simulink model "Machine_synchrone"  (R2016a)
settings: Solver=VariableStepAuto  StartTime=0.0  StopTime=0.3  RelTol=1e-3
values from neighbouring files (symbols this model uses):
  Kid = 3/(Td*kd)    (= 16502.7862857)    [Data.m]
  Kiq = 3/(Tq*kq)    (= 9368.0205239)    [Data.m]
  Pd = 3/kd    (= 38.6928)    [Data.m]
  Pq = 3/kq    (= 34.3565217391)    [Data.m]
libraries: cstblocks x2
settings Model: Creator=NAD  LastModifiedBy=NAD

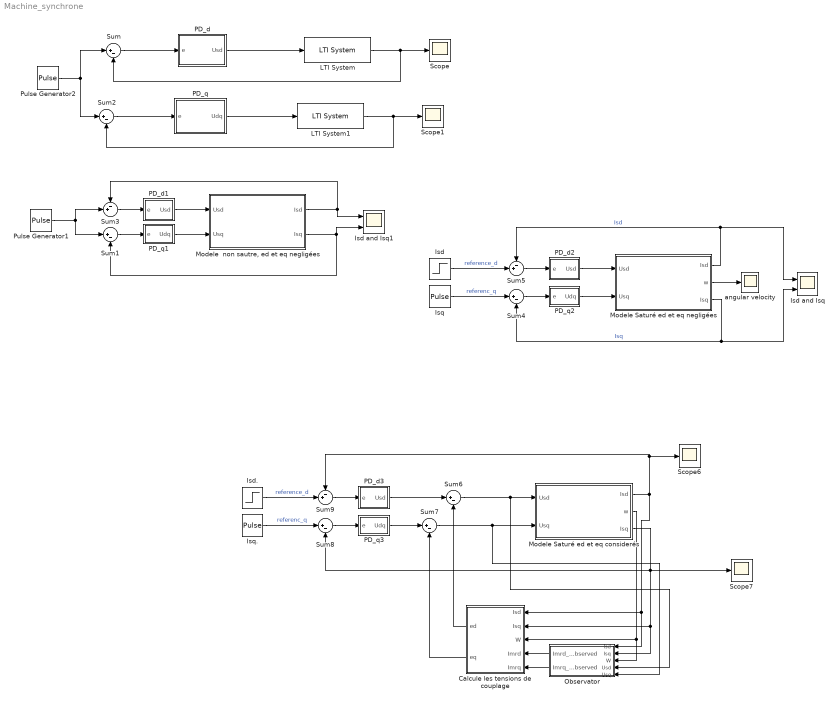
== system Machine_synchrone ==
  Calcule les tensions de couplage : MATLAB Function  TreatAsAtomicUnit=on
  Isd : Step  Time=0  After=10  SampleTime=0
  Isd and Isq : Scope  NumInputPorts=2
  Isd and Isq1 : Scope  NumInputPorts=2
  Isd. : Step  Time=0  After=10  SampleTime=0
  Isq : DiscretePulseGenerator  PulseType=Time based  Amplitude=10  Period=0.2  PulseWidth=50
  Isq. : DiscretePulseGenerator  PulseType=Time based  Amplitude=10  Period=0.2  PulseWidth=50
  LTI System : cstblocks/LTI System  sys=Fd  IC=[]
  LTI System1 : cstblocks/LTI System  sys=Fq  IC=[]
  "Modele  non sautre, ed et eq negligées" : Subsystem
  Modele Saturé ed et eq considerés : Subsystem
  Modele Saturé ed et eq negligées : Subsystem
  Observator : Subsystem
  PD_d : Subsystem
  PD_d1 : Subsystem
  PD_d2 : Subsystem
  PD_d3 : Subsystem
  PD_q : Subsystem
  PD_q1 : Subsystem
  PD_q2 : Subsystem
  PD_q3 : Subsystem
  Pulse Generator1 : DiscretePulseGenerator  PulseType=Time based  Amplitude=10  Period=1  PulseWidth=50
  Pulse Generator2 : DiscretePulseGenerator  PulseType=Time based  Amplitude=5  Period=0.01  PulseWidth=50
  Scope{,1,6..7} (4 alike) : Scope
  Sum{,1..2,4,6..8} (7 alike) : Sum  Inputs=|+-
  Sum3 : Sum  Inputs=-+|
  Sum5 : Sum  Inputs=-+|
  Sum9 : Sum  Inputs=-+|
  angular velocity : Scope
  wires:
  LTI System/1 -> Scope/1, Sum/2
  LTI System1/1 -> Scope1/1, Sum2/2
  Sum/1 -> PD_d/1(e)
  PD_d/1(Usd) -> LTI System/1
  Sum2/1 -> PD_q/1(e)
  PD_q/1(Udq) -> LTI System1/1
  PD_d1/1(Usd) -> "Modele  non sautre, ed et eq negligées"/1(Usd)
  PD_q1/1(Udq) -> "Modele  non sautre, ed et eq negligées"/2(Usq)
  "Modele  non sautre, ed et eq negligées"/1(Isd) -> Sum3/1, Isd and Isq1/1
  "Modele  non sautre, ed et eq negligées"/2(Isq) -> Sum1/2, Isd and Isq1/2
  Sum1/1 -> PD_q1/1(e)
  Sum3/1 -> PD_d1/1(e)
  Pulse Generator1/1 -> Sum3/2, Sum1/1
  PD_d2/1(Usd) -> Modele Saturé ed et eq negligées/1(Usd)
  PD_q2/1(Udq) -> Modele Saturé ed et eq negligées/2(Usq)
  Modele Saturé ed et eq negligées/1(Isd) -> Isd and Isq/1, Sum5/1  "Isd"
  Sum4/1 -> PD_q2/1(e)
  Sum5/1 -> PD_d2/1(e)
  Isq/1 -> Sum4/1  "referenc_q"
  Modele Saturé ed et eq negligées/3(Isq) -> Isd and Isq/2, Sum4/2  "Isq"
  Sum6/1 -> Observator/4(Usd), Modele Saturé ed et eq considerés/1(Usd)
  Sum7/1 -> Observator/5(Usq), Modele Saturé ed et eq considerés/2(Usq)
  Modele Saturé ed et eq considerés/1(Isd) -> Scope6/1, Sum9/1, Calcule les tensions de couplage/1(Isd), Observator/1(Isd)
  Sum8/1 -> PD_q3/1(e)
  Sum9/1 -> PD_d3/1(e)
  Modele Saturé ed et eq considerés/3(Isq) -> Calcule les tensions de couplage/2(Isq), Observator/2(Isq), Scope7/1, Sum8/2
  Observator/1(Imrd_Observed) -> Calcule les tensions de couplage/4(Imrd)
  Observator/2(Imrq_Observed) -> Calcule les tensions de couplage/5(Imrq)
  Modele Saturé ed et eq considerés/2(w) -> Calcule les tensions de couplage/3(W), Observator/3(W)
  Calcule les tensions de couplage/1(ed) -> Sum6/2
  Calcule les tensions de couplage/2(eq) -> Sum7/2
  PD_q3/1(Udq) -> Sum7/1
  PD_d3/1(Usd) -> Sum6/1
  Pulse Generator2/1 -> Sum/1, Sum2/1
  Modele Saturé ed et eq negligées/2(w) -> angular velocity/1
  Isd/1 -> Sum5/2  "reference_d"
  Isq./1 -> Sum8/1  "referenc_q"
  Isd./1 -> Sum9/2  "reference_d"

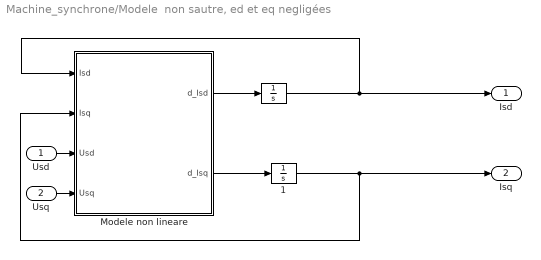
== system Machine_synchrone/Modele  non sautre, ed et eq negligées ==
  Usd : Inport
  Usq : Inport  Port=2
  " " : Integrator
  " 1" : Integrator
  Modele non lineare : MATLAB Function  TreatAsAtomicUnit=on
  Isd : Outport
  Isq : Outport  Port=2
  wires:
  Modele non lineare/2(d_Isq) -> " 1"/1
  " 1"/1 -> Isq/1, Modele non lineare/2(Isq)
  Usq/1 -> Modele non lineare/4(Usq)
  Usd/1 -> Modele non lineare/3(Usd)
  Modele non lineare/1(d_Isd) -> " "/1
  " "/1 -> Modele non lineare/1(Isd), Isd/1

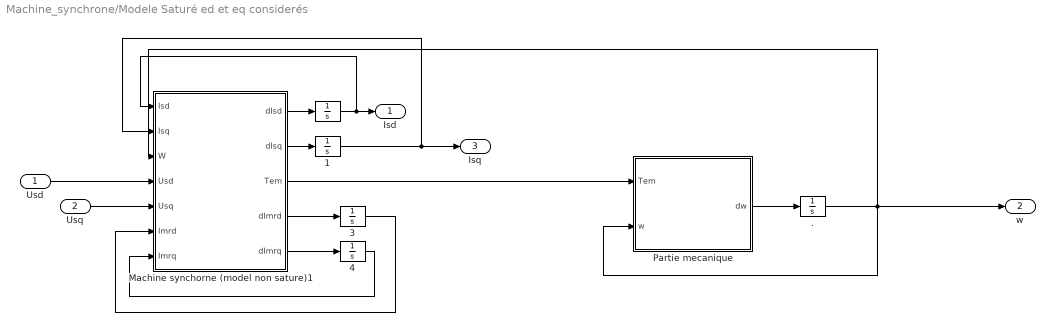
== system Machine_synchrone/Modele Saturé ed et eq considerés ==
  Usd : Inport
  Usq : Inport  Port=2
  " " : Integrator
  " ." : Integrator
  " 1" : Integrator
  " 3" : Integrator  InitialCondition=0.01
  " 4" : Integrator  InitialCondition=0.01
  Machine synchorne (model non sature)1 : MATLAB Function  TreatAsAtomicUnit=on
  Partie mecanique : MATLAB Function  TreatAsAtomicUnit=on
  Isd : Outport
  w : Outport  Port=2
  Isq : Outport  Port=3
  wires:
  " 3"/1 -> Machine synchorne (model non sature)1/6(Imrd)
  " 4"/1 -> Machine synchorne (model non sature)1/7(Imrq)
  Machine synchorne (model non sature)1/5(dImrq) -> " 4"/1
  Machine synchorne (model non sature)1/4(dImrd) -> " 3"/1
  Usq/1 -> Machine synchorne (model non sature)1/5(Usq)
  Usd/1 -> Machine synchorne (model non sature)1/4(Usd)
  " 1"/1 -> Isq/1, Machine synchorne (model non sature)1/2(Isq)
  Machine synchorne (model non sature)1/2(dIsq) -> " 1"/1
  Machine synchorne (model non sature)1/3(Tem) -> Partie mecanique/1(Tem)
  Partie mecanique/1(dw) -> " ."/1
  " ."/1 -> Machine synchorne (model non sature)1/3(W), Partie mecanique/2(w), w/1
  " "/1 -> Machine synchorne (model non sature)1/1(Isd), Isd/1
  Machine synchorne (model non sature)1/1(dIsd) -> " "/1

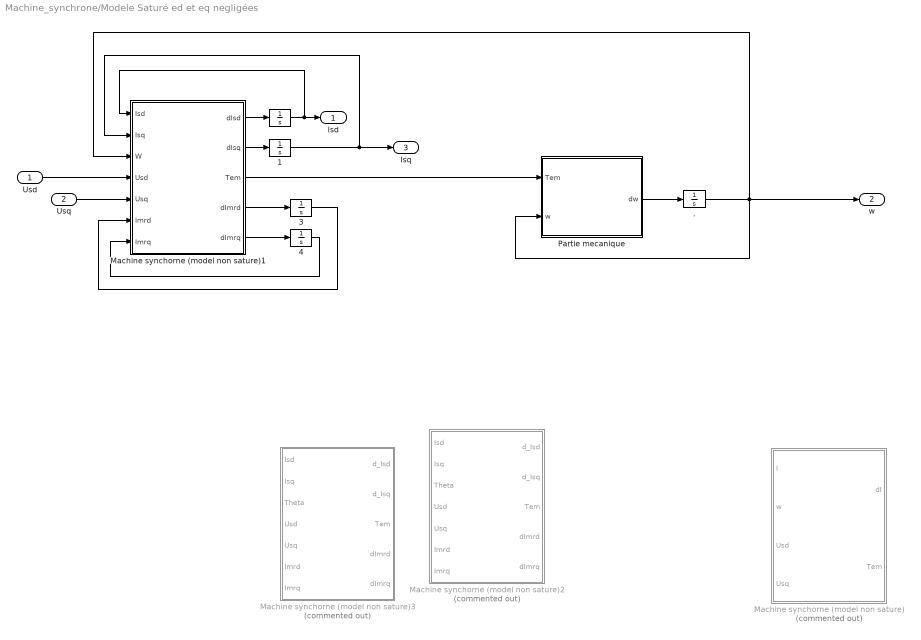
== system Machine_synchrone/Modele Saturé ed et eq negligées ==
  Usd : Inport
  Usq : Inport  Port=2
  " " : Integrator
  " ." : Integrator
  " 1" : Integrator
  " 3" : Integrator  InitialCondition=0.01
  " 4" : Integrator  InitialCondition=0.01
  Machine synchorne (model non sature) : MATLAB Function  Commented=on  TreatAsAtomicUnit=on
  Machine synchorne (model non sature)1 : MATLAB Function  TreatAsAtomicUnit=on
  Machine synchorne (model non sature)2 : MATLAB Function  Commented=on  TreatAsAtomicUnit=on
  Machine synchorne (model non sature)3 : MATLAB Function  Commented=on  TreatAsAtomicUnit=on
  Partie mecanique : MATLAB Function  TreatAsAtomicUnit=on
  Isd : Outport
  w : Outport  Port=2
  Isq : Outport  Port=3
  wires:
  Machine synchorne (model non sature)1/1(dIsd) -> " "/1
  " "/1 -> Isd/1, Machine synchorne (model non sature)1/1(Isd)
  " ."/1 -> w/1, Partie mecanique/2(w), Machine synchorne (model non sature)1/3(W)
  Partie mecanique/1(dw) -> " ."/1
  Machine synchorne (model non sature)1/3(Tem) -> Partie mecanique/1(Tem)
  Machine synchorne (model non sature)1/2(dIsq) -> " 1"/1
  " 1"/1 -> Machine synchorne (model non sature)1/2(Isq), Isq/1
  Usd/1 -> Machine synchorne (model non sature)1/4(Usd)
  Usq/1 -> Machine synchorne (model non sature)1/5(Usq)
  Machine synchorne (model non sature)1/4(dImrd) -> " 3"/1
  Machine synchorne (model non sature)1/5(dImrq) -> " 4"/1
  " 4"/1 -> Machine synchorne (model non sature)1/7(Imrq)
  " 3"/1 -> Machine synchorne (model non sature)1/6(Imrd)

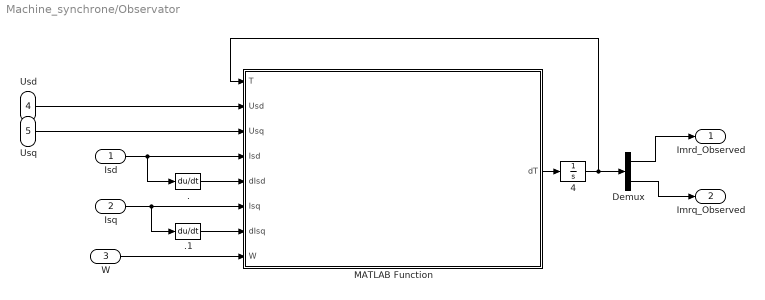
== system Machine_synchrone/Observator ==
  Isd : Inport
  Isq : Inport  Port=2
  W : Inport  Port=3
  Usd : Inport  Port=4
  Usq : Inport  Port=5
  " 4" : Integrator  InitialCondition=0.01*[1;1]
  . : Derivative
  .1 : Derivative
  Demux : Demux  Outputs=2
  MATLAB Function : MATLAB Function  TreatAsAtomicUnit=on
  Imrd_Observed : Outport
  Imrq_Observed : Outport  Port=2
  wires:
  W/1 -> MATLAB Function/8(W)
  .1/1 -> MATLAB Function/7(dIsq)
  MATLAB Function/1(dT) -> " 4"/1
  " 4"/1 -> Demux/1, MATLAB Function/1(T)
  ./1 -> MATLAB Function/5(dIsd)
  Demux/1 -> Imrd_Observed/1
  Isq/1 -> .1/1, MATLAB Function/6(Isq)
  Isd/1 -> MATLAB Function/4(Isd), ./1
  Usd/1 -> MATLAB Function/2(Usd)
  Demux/2 -> Imrq_Observed/1
  Usq/1 -> MATLAB Function/3(Usq)

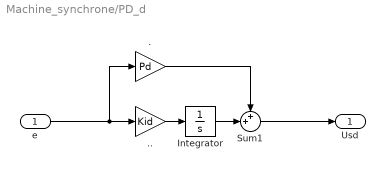
== system Machine_synchrone/PD_d ==
  e : Inport
  ". " : Gain  Gain=Pd
  .. : Gain  Gain=Kid
  Integrator : Integrator
  Sum1 : Sum  Inputs=++|
  Usd : Outport
  wires:
  Sum1/1 -> Usd/1
  e/1 -> ../1, ". "/1
  ". "/1 -> Sum1/1
  Integrator/1 -> Sum1/2
  ../1 -> Integrator/1

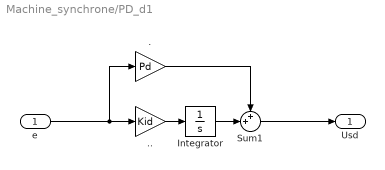
== system Machine_synchrone/PD_d1 ==
  e : Inport
  ". " : Gain  Gain=Pd
  .. : Gain  Gain=Kid
  Integrator : Integrator
  Sum1 : Sum  Inputs=++|
  Usd : Outport
  wires:
  ../1 -> Integrator/1
  Integrator/1 -> Sum1/2
  ". "/1 -> Sum1/1
  e/1 -> ". "/1, ../1
  Sum1/1 -> Usd/1

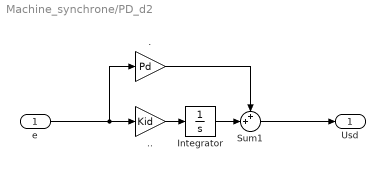
== system Machine_synchrone/PD_d2 ==
  e : Inport
  ". " : Gain  Gain=Pd
  .. : Gain  Gain=Kid
  Integrator : Integrator
  Sum1 : Sum  Inputs=++|
  Usd : Outport
  wires:
  ../1 -> Integrator/1
  Integrator/1 -> Sum1/2
  ". "/1 -> Sum1/1
  e/1 -> ". "/1, ../1
  Sum1/1 -> Usd/1

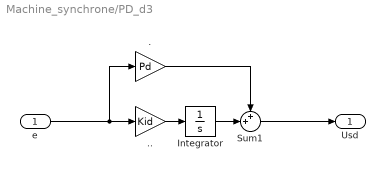
== system Machine_synchrone/PD_d3 ==
  e : Inport
  ". " : Gain  Gain=Pd
  .. : Gain  Gain=Kid
  Integrator : Integrator
  Sum1 : Sum  Inputs=++|
  Usd : Outport
  wires:
  Sum1/1 -> Usd/1
  e/1 -> ../1, ". "/1
  ". "/1 -> Sum1/1
  Integrator/1 -> Sum1/2
  ../1 -> Integrator/1

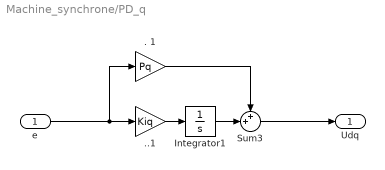
== system Machine_synchrone/PD_q ==
  e : Inport
  . 1 : Gain  Gain=Pq
  ..1 : Gain  Gain=Kiq
  Integrator1 : Integrator
  Sum3 : Sum  Inputs=++|
  Udq : Outport
  wires:
  Sum3/1 -> Udq/1
  Integrator1/1 -> Sum3/2
  . 1/1 -> Sum3/1
  e/1 -> . 1/1, ..1/1
  ..1/1 -> Integrator1/1

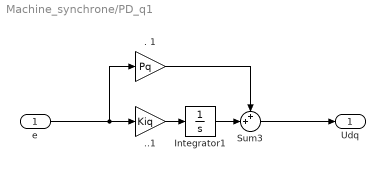
== system Machine_synchrone/PD_q1 ==
  e : Inport
  . 1 : Gain  Gain=Pq
  ..1 : Gain  Gain=Kiq
  Integrator1 : Integrator
  Sum3 : Sum  Inputs=++|
  Udq : Outport
  wires:
  ..1/1 -> Integrator1/1
  e/1 -> ..1/1, . 1/1
  . 1/1 -> Sum3/1
  Integrator1/1 -> Sum3/2
  Sum3/1 -> Udq/1

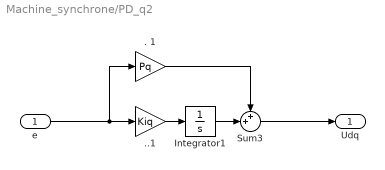
== system Machine_synchrone/PD_q2 ==
  e : Inport
  . 1 : Gain  Gain=Pq
  ..1 : Gain  Gain=Kiq
  Integrator1 : Integrator
  Sum3 : Sum  Inputs=++|
  Udq : Outport
  wires:
  ..1/1 -> Integrator1/1
  e/1 -> ..1/1, . 1/1
  . 1/1 -> Sum3/1
  Integrator1/1 -> Sum3/2
  Sum3/1 -> Udq/1

== system Machine_synchrone/PD_q3 ==
  e : Inport
  . 1 : Gain  Gain=Pq
  ..1 : Gain  Gain=Kiq
  Integrator1 : Integrator
  Sum3 : Sum  Inputs=++|
  Udq : Outport
  wires:
  Sum3/1 -> Udq/1
  Integrator1/1 -> Sum3/2
  . 1/1 -> Sum3/1
  e/1 -> . 1/1, ..1/1
  ..1/1 -> Integrator1/1

== matlab function Machine_synchrone/Modele Saturé ed et eq negligées/Machine synchorne (model non sature) ==
  data: I input; w input; Usd input; Usq input; dI output; Tem output
function [dI , Tem]= fct(I,w,Usd,Usq)
%% Les parametres:
Rs=7.8;
Ld = 0.54 ;
wd=0.056;
Trd =0.1;
Lq=0.21;
wq=0.2;
Trq=0.046;

kd =1/(Rs+Ld*(1-wd)/Trd); Td = wd*Ld*kd;
kq =1/(Rs+Lq*(1-wq)/Trq); Tq = wq*Lq*kq;
% Paramatres supposés :
Lrd = Ld/3; Rrd = 1.97; Md = 0.33 ;
Lrq = 0.07; Rrq = 0.346; Mq = 0.13 ;
p = 3; 
% la vitesse angulaire electrique:
we = p*w;
% le vecteurs et matrices d'etat:
U = [Usd,Usq,0,0]';
W = [0, -we ; we, 0];
RRs = [Rs , 0; 0, Rs];
RRr = [Rrd, 0; 0, Rrq];
Ls = [Ld, 0 ; 0, Lq];
Lr = [Lrd, 0 ; 0, Lrq];
M = [Md, 0; 0, Mq]*0;
R = [RRs+W*Ls, W*M; zeros(2,2), RRr];
L = [Ls, M; M, Lr];

%% le systeme 
% U = RI + LdI;
dI = L\(U-R*I);
% Us=[Usd;Usq];
% Is=I(1:2); Ir=I(3:4);
% dIs = (Ls-M*Lr\M)\(Us-(RRs+W*Ls)*Is+(W*M-M*RRr/Lr)*Ir );
% dIr = -Lr\RRr*Ir-Lr\M*dIs;
% dI=[dIs;dIr];
isd = dI(1); isq = dI(2);
Tem = p*(Ld-Lq)*isd*isq;

== matlab function Machine_synchrone/Modele  non sautre, ed et eq negligées/Modele non lineare ==
  data: Isd input; d_Isd output; Isq input; Usd input; Usq input; d_Isq output
function [d_Isd,d_Isq] = fct(Isd,Isq,Usd,Usq)
% Les parametres:
Rs =7.8;
Ld = 0.54 ;
wd=0.056;
Trd =0.1;
Lq=0.21;
wq=0.2;
Trq=0.046;

kd =1/(Rs+Ld*(1-wd)/Trd); Td = wd*Ld*kd;
kq =1/(Rs+Lq*(1-wq)/Trq); Tq = wq*Lq*kq;

% le systeme 
d_Isd = -1/Td*Isd + (Usd)/ (wd*Ld);
d_Isq = -1/Tq*Isq + (Usq)/(wq*Lq);

== matlab function Machine_synchrone/Modele Saturé ed et eq negligées/Machine synchorne (model non sature)1 ==
  data: Isd input; Isq input; W input; Usd input; Usq input; dIsd output; dIsq output; Tem output; Imrd input; Imrq input; dImrd output; dImrq output
function [dIsd,dIsq,Tem,dImrd,dImrq] = fct(Isd,Isq,W,Usd,Usq,Imrd,Imrq)
%% Les parametres:
Rs=7.8;
Ld = 0.54 ;
wd=0.056;
Trd =0.1;
Lq=0.21;
wq=0.2;
Trq=0.046;

% Paramatres supposés :
p = 3; 
% la vitesse angulaire electrique:
we=p*W;
% le coeficient de transformation du champ magentique Imr d'une machine a poles saillants vers un chemp magnetisant magnetisant equivalent Imr_ d'une magine a pole sille
k=sqrt(Lq*(1-wq)/Ld/(1-wd));
% Le champs magnetisant equivalent:
Imr_ = sqrt(Imrd^2+Imrq^2*k^2);
% le coefficient de saturation Ks(Imr_) = N/D
a = -1.376 ; c =-0.0247 ; e= -1.381 ; g=-0.080;
b= 0.586 ; d= 0.005 ; f =0.619 ; h =0.033;
N = 1 + a*Imr_ + b*Imr_^2 + c*Imr_^3 + d*Imr_^4;
D = 1 + e*Imr_ + f*Imr_^2 + g*Imr_^3 + h*Imr_^4;
Ks = N/D;
% le coefficient de saturation dynamique Ksd(Imr_) = dKs/dImr_ 
dN = a + 2*b*Imr_ + 3*c*Imr_^2 + 4*d*Imr_^3;
dD = e + 2*f*Imr_ + 3*g*Imr_^2 + 4*h*Imr_^3;
Ksd = (dN*D-dD*N)/D^2;
% Ks= 1; Ksd =0.005;
% autre coefficients d'induction:
Ldd = Ld*(1-wd)*(Ks+Ksd*Imrd^2/Imr_);
Lqq = Lq*(1-wq)*(Ks+k^2*Ksd*Imrq^2/Imr_);
Mdq = Lq*(1-wq)*Ksd*Imrd*Imrq/Imr_;


%% le systeme 
% Les parametres de la matrce:
a1 = -(Rs/wd/Ld+(1-wd)/wd/Trd);b1= we*wq*Lq/wd/Ld; c1=(1-wd)/wd/Trd ;d1= Ks*we*Lq*(1-wq)/wd/Ld ; e1=1/(wd*Ld) ;
a2 =- we*wd*Ld/wq/Lq ;b2=-(Rs/wq/Lq+(1-wq)/wq/Trq) ; c2=- Ks*we*Ld*(1-wd)/wq/Lq ;d2= (1-wq)/wq/Trq; e2=1/(wq*Lq) ;
a3 = 1/(Ks*(Ks+Ksd*Imr_))*(Lqq/Trd/Lq/(1-wq)) ;b3= -1/(Ks*(Ks+Ksd*Imr_))*k^2*Mdq/Trq/Lq/(1-wq) ; c3= -a3; d3= -b3 ; 
a4 = -1/(Ks*(Ks+Ksd*Imr_))*Mdq/Trd/Lq/(1-wq);b4= 1/(Ks*(Ks+Ksd*Imr_))*(Ldd/Trq/Ld/(1-wd)); c4=-a4 ;d4=-b4 ; 

I=[Isd;Isq;Imrd;Imrq]; U = [Usd;Usq]; 
A= [a1 b1 c1 d1
    a2 b2 c2 d2
    a3 b3 c3 d3
    a4 b4 c4 d4];
B= [e1 0
    0 e2
    0 0
    0 0];
dI = A*I+B*U;
dIsd = dI(1);
dIsq = dI(2);
dImrd = dI(3);
dImrq = dI(4);

Tem = p*(Ld-Lq)*Isd*Isq;

% % les equations de courants statoriques:
% dIsd = -(Rs/wd/Ld+(1-wd)/wd/Trd)*Isd + we*wq*Lq/wd/Ld*Isq+(1-wd)/wd/Trd*Imrd + Ks*we*Lq*(1-wq)/wd/Ld*Imrq + 1/(wd*Ld)*Usd;
% dIsq = -(Rs/wq/Lq+(1-wq)/wq/Trq)*Isq - we*wd*Ld/wq/Lq*Isd+(1-wq)/wq/Trq*Imrq - Ks*we*Ld*(1-wd)/wq/Lq*Imrd + 1/(wq*Lq)*Usq;
% 
% % le courants de magnetisation:
% dImrd = 1/(Ks*(Ks+Ksd*Imr_))*(Lqq/Trd/Lq/(1-wq)*(Isd-Imrd)+k^2*Mdq/Trq/Lq/(1-wq)*(Imrq-Isq));
% dImrq = 1/(Ks*(Ks+Ksd*Imr_))*(Ldd/Trq/Ld/(1-wd)*(Isq-Imrq)+ Mdq/Trd/Lq/(1-wq)*(Imrd-Isd));
% 

% 
% 
% Imrd= Isd + Lrd/Md*ird;
% Imrq = Isq + Lrq/Md*irq;

== matlab function Machine_synchrone/Modele Saturé ed et eq negligées/Machine synchorne (model non sature)2 ==
  data: Isd input; Isq input; Theta input; Usd input; Usq input; d_Isd output; d_Isq output; Tem output; Imrd input; Imrq input; dImrd output; dImrq output
function [d_Isd,d_Isq,Tem,dImrd,dImrq] = fct(Isd,Isq,Theta,Usd,Usq,Imrd,Imrq)
%% Les parametres:
Rs=7.8;
Ld = 0.54 ;
wd=0.056;
Trd =0.1;
Lq=0.21;
wq=0.2;
Trq=0.046;

kd =1/(Rs+Ld*(1-wd)/Trd); Td = wd*Ld*kd;
kq =1/(Rs+Lq*(1-wq)/Trq); Tq = wq*Lq*kq;
% Paramatres supposés :
p = 3; 
% la vitesse angulaire electrique:
we=p*Theta;
% le coeficient de transformation du champ magentique Imr d'une machine a poles saillants vers un chemp magnetisant magnetisant equivalent Imr_ d'une magine a pole sille
k=sqrt(Lq*(1-wq)/Ld/(1-wd));
% Le champs magnetisant equivalent:
Imr_ = sqrt(Imrd^2+Imrq^2*k^2);
% le coefficient de saturation Ks(Imr_) = N/D
a = -1.376 ; c =-0.0247 ; e= -1.381 ; g=-0.080;
b= 0.586 ; d= 0.005 ; f =0.619 ; h =0.033;
N = 1 + a*Imr_ + b*Imr_^2 + c*Imr_^3 + d*Imr_^4;
D = 1 + e*Imr_ + f*Imr_^2 + g*Imr_^3 + h*Imr_^4;
Ks = N/D;
% le coefficient de saturation dynamique Ksd(Imr_) = dKs/dImr_ 
dN = a + 2*b*Imr_ + 3*c*Imr_^2 + 4*d*Imr_^3;
dD = e + 2*f*Imr_ + 3*g*Imr_^2 + 4*h*Imr_^3;
Ksd = (dN*D-dD*N)/D^2;
% autre coefficients d'induction:
Ldd = Ld*(1-wd)*(Ks+Ksd*Imrd^2/Imr_);
Lqq = Lq*(1-wq)*(Ks+k^2*Ksd*Imrq^2/Imr_);
Mdq = Lq*(1-wq)*Ksd*Imrd*Imrq/Imr_;


%% le systeme 
% le courants de magnetisation:
dImrd = 1/(Ks*(Ks+Ksd*Imr_))*(Lqq/Trd/Lq/(1-wq)*(Isd-Imrd)+k^2*Mdq/Trq/Lq/(1-wq)*(Imrq-Isq));
dImrq = 1/(Ks*(Ks+Ksd*Imr_))*(Ldd/Trq/Ld/(1-wd)*(Isq-Imrq)+ Mdq/Trd/Lq/(1-wq)*(Imrd-Isd));

% les tensions de couplages
ed = we*(wq*Lq*Isq + Lq*(1-wq)*Imrq) + Ld*(1-wd)/Trd*Imrd;
eq = -we*(wd*Ld*Isd + Ld*(1-wd)*Imrd) + Lq*(1-wq)/Trq*Imrq;
% les equations de courants statoriques:
d_Isd = -1/Td*Isd + (Usd+ed)/ (wd*Ld);
d_Isq = -1/Tq*Isq + (Usq+eq)/(wq*Lq);

Tem = p*(Ld-Lq)*Isd*Isq;


% 
% 
% Imrd= Isd + Lrd/Md*ird;
% Imrq = Isq + Lrq/Md*irq;

== matlab function Machine_synchrone/Modele Saturé ed et eq negligées/Machine synchorne (model non sature)3 ==
  data: Isd input; Isq input; Theta input; Usd input; Usq input; d_Isd output; d_Isq output; Tem output; Imrd input; Imrq input; dImrd output; dImrq output
function [d_Isd,d_Isq,Tem,dImrd,dImrq] = fct(Isd,Isq,Theta,Usd,Usq,Imrd,Imrq)
%% Les parametres:
Rs=7.8;
Ld = 0.54 ;
wd=0.056;
Trd =0.1;
Lq=0.21;
wq=0.2;
Trq=0.046;

kd =1/(Rs+Ld*(1-wd)/Trd); Td = wd*Ld*kd;
kq =1/(Rs+Lq*(1-wq)/Trq); Tq = wq*Lq*kq;
% Paramatres supposés :
p = 3; 
% la vitesse angulaire electrique:
we=p*Theta;
% le coeficient de transformation du champ magentique Imr d'une machine a poles saillants vers un chemp magnetisant magnetisant equivalent Imr_ d'une magine a pole sille
k=sqrt(Lq*(1-wq)/Ld/(1-wd));
% Le champs magnetisant equivalent:
Imr_ = sqrt(Imrd^2+Imrq^2*k^2);
% le coefficient de saturation Ks(Imr_) = N/D
a = -1.376 ; c =-0.0247 ; e= -1.381 ; g=-0.080;
b= 0.586 ; d= 0.005 ; f =0.619 ; h =0.033;
N = 1 + a*Imr_ + b*Imr_^2 + c*Imr_^3 + d*Imr_^4;
D = 1 + e*Imr_ + f*Imr_^2 + g*Imr_^3 + h*Imr_^4;
Ks = N/D;
% le coefficient de saturation dynamique Ksd(Imr_) = dKs/dImr_ 
dN = a + 2*b*Imr_ + 3*c*Imr_^2 + 4*d*Imr_^3;
dD = e + 2*f*Imr_ + 3*g*Imr_^2 + 4*h*Imr_^3;
Ksd = (dN*D-dD*N)/D^2;
% autre coefficients d'induction:
Ldd = Ld*(1-wd)*(Ks+Ksd*Imrd^2/Imr_);
Lqq = Lq*(1-wq)*(Ks+k^2*Ksd*Imrq^2/Imr_);
Mdq = Lq*(1-wq)*Ksd*Imrd*Imrq/Imr_;


%% le systeme 
% Les parametres de la matrce:
% le courants de magnetisation:
dImrd = 1/(Ks*(Ks+Ksd*Imr_))*(Lqq/Trd/Lq/(1-wq)*(Isd-Imrd)+k^2*Mdq/Trq/Lq/(1-wq)*(Imrq-Isq));
dImrq = 1/(Ks*(Ks+Ksd*Imr_))*(Ldd/Trq/Ld/(1-wd)*(Isq-Imrq)+ Mdq/Trd/Lq/(1-wq)*(Imrd-Isd));

% les equations de courants statoriques:
d_Isd = -(Rs/wd/Ld+(1-wd)/wd/Trd)*Isd + we*wq*Lq/wd/Ld*Isq+(1-wd)/wd/Trd*Imrd + Ks*we*Lq*(1-wq)/wd/Ld*Imrq + 1/(wd*Ld)*Usd;
d_Isq = -(Rs/wq/Lq+(1-wq)/wq/Trq)*Isq - we*wd*Ld/wq/Lq*Isd+(1-wq)/wq/Trq*Imrq - Ks*we*Ld*(1-wd)/wq/Lq*Imrd + 1/(wq*Lq)*Usq;

Tem = p*(Ld-Lq)*Isd*Isq;


% 
% 
% Imrd= Isd + Lrd/Md*ird;
% Imrq = Isq + Lrq/Md*irq;

== matlab function Machine_synchrone/Modele Saturé ed et eq negligées/Partie mecanique ==
  data: Tem input; w input; dw output
function dw  = fct(Tem,w)
%% Les parametres:
J = 0.05;
f = 0.002 ;

dw= -f/J*w + Tem/J;

== matlab function Machine_synchrone/Calcule les tensions de couplage ==
  data: Isd input; ed output; Isq input; W input; Imrd input; Imrq input; eq output
function [ed,eq] = fct(Isd,Isq,W,Imrd,Imrq)
%% Les parametres:
Rs=7.8;
Ld = 0.54 ;
wd=0.056;
Trd =0.1;
Lq=0.21;
wq=0.2;
Trq=0.046;

% Paramatres supposés :
p = 3; 
% la vitesse angulaire electrique:
we=p*W;
% le coeficient de transformation du champ magentique Imr d'une machine a poles saillants vers un chemp magnetisant magnetisant equivalent Imr_ d'une magine a pole sille
k=sqrt(Lq*(1-wq)/Ld/(1-wd));
% Le champs magnetisant equivalent:
Imr_ = sqrt(Imrd^2+Imrq^2*k^2);
% le coefficient de saturation Ks(Imr_) = N/D
a = -1.376 ; c =-0.0247 ; e= -1.381 ; g=-0.080;
b= 0.586 ; d= 0.005 ; f =0.619 ; h =0.033;
N = 1 + a*Imr_ + b*Imr_^2 + c*Imr_^3 + d*Imr_^4;
D = 1 + e*Imr_ + f*Imr_^2 + g*Imr_^3 + h*Imr_^4;
Ks = N/D;
%%

% les tensions de couplages
ed = we*(wq*Lq*Isq + Lq*(1-wq)*Imrq) + Ld*(1-wd)/Trd*Imrd;
eq = -we*(wd*Ld*Isd + Ld*(1-wd)*Imrd) + Lq*(1-wq)/Trq*Imrq;

== matlab function Machine_synchrone/Observator/MATLAB Function ==
  data: T input; dT output; Usd input; Usq input; Isd input; dIsd input; Isq input; dIsq input; W input
function dT = fct(T,Usd,Usq,Isd,dIsd,Isq,dIsq,W)
%% Les parametres:
Rs=7.8;
Ld = 0.54 ;
wd=0.056;
Trd =0.1;
Lq=0.21;
wq=0.2;
Trq=0.046;

% Paramatres supposés :
p = 3; 
% la vitesse angulaire electrique:
we=p*W;
% le coeficient de transformation du champ magentique Imr d'une machine a poles saillants vers un chemp magnetisant magnetisant equivalent Imr_ d'une magine a pole sille
k=sqrt(Lq*(1-wq)/Ld/(1-wd));
% Le champs magnetisant equivalent:
Imrd = T(1); Imrq=T(2);
Imr_ = sqrt(Imrd^2+Imrq^2*k^2);
% le coefficient de saturation Ks(Imr_) = N/D
a = -1.376 ; c =-0.0247 ; e= -1.381 ; g=-0.080;
b= 0.586 ; d= 0.005 ; f =0.619 ; h =0.033;
N = 1 + a*Imr_ + b*Imr_^2 + c*Imr_^3 + d*Imr_^4;
D = 1 + e*Imr_ + f*Imr_^2 + g*Imr_^3 + h*Imr_^4;
Ks = N/D;
% le coefficient de saturation dynamique Ksd(Imr_) = dKs/dImr_ 
dN = a + 2*b*Imr_ + 3*c*Imr_^2 + 4*d*Imr_^3;
dD = e + 2*f*Imr_ + 3*g*Imr_^2 + 4*h*Imr_^3;
Ksd = (dN*D-dD*N)/D^2;
% Ks= 1; Ksd =0.005;
% autre coefficients d'induction:
Ldd = Ld*(1-wd)*(Ks+Ksd*Imrd^2/Imr_);
Lqq = Lq*(1-wq)*(Ks+k^2*Ksd*Imrq^2/Imr_);
Mdq = Lq*(1-wq)*Ksd*Imrd*Imrq/Imr_;


%% le systeme 
% Les parametres de la matrce:
a1 = -(Rs/wd/Ld+(1-wd)/wd/Trd);b1= we*wq*Lq/wd/Ld; c1=(1-wd)/wd/Trd ;d1= Ks*we*Lq*(1-wq)/wd/Ld ; e1=1/(wd*Ld) ;
a2 =- we*wd*Ld/wq/Lq ;b2=-(Rs/wq/Lq+(1-wq)/wq/Trq) ; c2=- Ks*we*Ld*(1-wd)/wq/Lq ;d2= (1-wq)/wq/Trq; e2=1/(wq*Lq) ;
a3 = 1/(Ks*(Ks+Ksd*Imr_))*(Lqq/Trd/Lq/(1-wq)) ;b3= -1/(Ks*(Ks+Ksd*Imr_))*k^2*Mdq/Trq/Lq/(1-wq) ; c3= -a3; d3= -b3 ; 
a4 = -1/(Ks*(Ks+Ksd*Imr_))*Mdq/Trd/Lq/(1-wq);b4= 1/(Ks*(Ks+Ksd*Imr_))*(Ldd/Trq/Ld/(1-wd)); c4=-a4 ;d4=-b4 ; 


%%
Is = [Isd;Isq];
dIs = [dIsd;dIsq];
Us = [Usd;Usq];

Um = [a3 b3; a4 b4]*Is;
Ym = [c1 d1; c2 d2]\(dIs-[a1 b1; a2 b2]*Is-[e1 0 ;0 e2]*Us);
Am = [c3 d3; c4 d4];

l = 50;
Km = Am + [l 0; 0 l];
dT = -[l 0; 0 l]*T + Um + Km*Ym;

== matlab function Machine_synchrone/Modele Saturé ed et eq considerés/Machine synchorne (model non sature)1 ==
  data: Isd input; Isq input; W input; Usd input; Usq input; dIsd output; dIsq output; Tem output; Imrd input; Imrq input; dImrd output; dImrq output
function [dIsd,dIsq,Tem,dImrd,dImrq] = fct(Isd,Isq,W,Usd,Usq,Imrd,Imrq)
%% Les parametres:
Rs=7.8;
Ld = 0.54 ;
wd=0.056;
Trd =0.1;
Lq=0.21;
wq=0.2;
Trq=0.046;

% Paramatres supposés :
p = 3; 
% la vitesse angulaire electrique:
we=p*W;
% le coeficient de transformation du champ magentique Imr d'une machine a poles saillants vers un chemp magnetisant magnetisant equivalent Imr_ d'une magine a pole sille
k=sqrt(Lq*(1-wq)/Ld/(1-wd));
% Le champs magnetisant equivalent:
Imr_ = sqrt(Imrd^2+Imrq^2*k^2);
% le coefficient de saturation Ks(Imr_) = N/D
a = -1.376 ; c =-0.0247 ; e= -1.381 ; g=-0.080;
b= 0.586 ; d= 0.005 ; f =0.619 ; h =0.033;
N = 1 + a*Imr_ + b*Imr_^2 + c*Imr_^3 + d*Imr_^4;
D = 1 + e*Imr_ + f*Imr_^2 + g*Imr_^3 + h*Imr_^4;
Ks = N/D;
% le coefficient de saturation dynamique Ksd(Imr_) = dKs/dImr_      
dN = a + 2*b*Imr_ + 3*c*Imr_^2 + 4*d*Imr_^3;
dD = e + 2*f*Imr_ + 3*g*Imr_^2 + 4*h*Imr_^3;
Ksd = (dN*D-dD*N)/D^2;
% Ks= 1; Ksd =0.005;
% autre coefficients d'induction:
Ldd = Ld*(1-wd)*(Ks+Ksd*Imrd^2/Imr_);
Lqq = Lq*(1-wq)*(Ks+k^2*Ksd*Imrq^2/Imr_);
Mdq = Lq*(1-wq)*Ksd*Imrd*Imrq/Imr_;


%% le systeme 
% Les parametres de la matrce:
a1 = -(Rs/wd/Ld+(1-wd)/wd/Trd);b1= we*wq*Lq/wd/Ld; c1=(1-wd)/wd/Trd ;d1= Ks*we*Lq*(1-wq)/wd/Ld ; e1=1/(wd*Ld) ;
a2 =- we*wd*Ld/wq/Lq ;b2=-(Rs/wq/Lq+(1-wq)/wq/Trq) ; c2=- Ks*we*Ld*(1-wd)/wq/Lq ;d2= (1-wq)/wq/Trq; e2=1/(wq*Lq) ;
a3 = 1/(Ks*(Ks+Ksd*Imr_))*(Lqq/Trd/Lq/(1-wq)) ;b3= -1/(Ks*(Ks+Ksd*Imr_))*k^2*Mdq/Trq/Lq/(1-wq) ; c3= -a3; d3= -b3 ; 
a4 = -1/(Ks*(Ks+Ksd*Imr_))*Mdq/Trd/Lq/(1-wq);b4= 1/(Ks*(Ks+Ksd*Imr_))*(Ldd/Trq/Ld/(1-wd)); c4=-a4 ;d4=-b4 ; 

I=[Isd;Isq;Imrd;Imrq]; U = [Usd;Usq]; 
A= [a1 b1 c1 d1
    a2 b2 c2 d2
    a3 b3 c3 d3
    a4 b4 c4 d4];
B= [e1 0
    0 e2
    0 0
    0 0];
dI = A*I+B*U;
dIsd = dI(1);
dIsq = dI(2);
dImrd = dI(3);
dImrq = dI(4);

Tem = p*(Ld-Lq)*Isd*Isq;

% % les equations de courants statoriques:
% dIsd = -(Rs/wd/Ld+(1-wd)/wd/Trd)*Isd + we*wq*Lq/wd/Ld*Isq+(1-wd)/wd/Trd*Imrd + Ks*we*Lq*(1-wq)/wd/Ld*Imrq + 1/(wd*Ld)*Usd;
% dIsq = -(Rs/wq/Lq+(1-wq)/wq/Trq)*Isq - we*wd*Ld/wq/Lq*Isd+(1-wq)/wq/Trq*Imrq - Ks*we*Ld*(1-wd)/wq/Lq*Imrd + 1/(wq*Lq)*Usq;
% 
% % le courants de magnetisation:
% dImrd = 1/(Ks*(Ks+Ksd*Imr_))*(Lqq/Trd/Lq/(1-wq)*(Isd-Imrd)+k^2*Mdq/Trq/Lq/(1-wq)*(Imrq-Isq));
% dImrq = 1/(Ks*(Ks+Ksd*Imr_))*(Ldd/Trq/Ld/(1-wd)*(Isq-Imrq)+ Mdq/Trd/Lq/(1-wq)*(Imrd-Isd));
% 

% 
% 
% Imrd= Isd + Lrd/Md*ird;
% Imrq = Isq + Lrq/Md*irq;

== matlab function Machine_synchrone/Modele Saturé ed et eq considerés/Partie mecanique ==
  data: Tem input; w input; dw output
function dw  = fct(Tem,w)
%% Les parametres:
J = 50;
f = 0.01 ;

dw= -f/J*w + Tem/J;
